simulink model "test_3_un_tanque_nivel_incicial_distinto_de_0_r2016a"  (R2016a)
settings: Solver=ode23tb  StartTime=0.0  StopTime=5.0  RelTol=1e-3
settings Model: Creator=Matias  LastModifiedBy=Matias

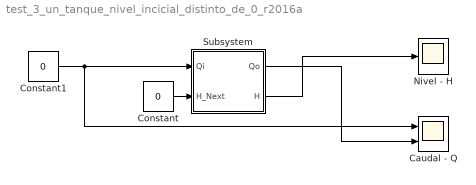
== system test_3_un_tanque_nivel_incicial_distinto_de_0_r2016a ==
  Caudal - Q : Scope  NumInputPorts=2
  Constant : Constant  Value=0
  Constant1 : Constant  Value=0
  Nivel - H : Scope
  Subsystem : Subsystem
  wires:
  Constant/1 -> Subsystem/2(H_Next)
  Constant1/1 -> Subsystem/1("Qi "), Caudal - Q/1
  Subsystem/1(Qo) -> Caudal - Q/2
  Subsystem/2("H ") -> Nivel - H/1

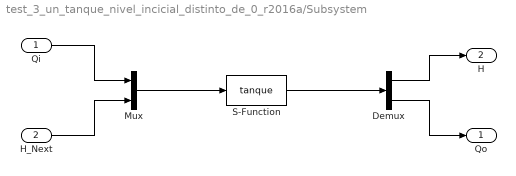
== system test_3_un_tanque_nivel_incicial_distinto_de_0_r2016a/Subsystem ==
  "Qi " : Inport
  H_Next : Inport  Port=2
  Demux : Demux  Outputs=2
  Mux : Mux  Inputs=2
  S-Function : S-Function  FunctionName=tanque  Parameters=1, 0.6, 1, 1  SFunctionDeploymentMode=off  EnableBusSupport=off
  Qo : Outport
  "H " : Outport  Port=2
  wires:
  Mux/1 -> S-Function/1
  "Qi "/1 -> Mux/1
  H_Next/1 -> Mux/2
  S-Function/1 -> Demux/1
  Demux/1 -> "H "/1
  Demux/2 -> Qo/1
